simulink model "motorC"  (R2017b)
settings: Solver=FixedStepAuto  StartTime=0.0  StopTime=60  FixedStep=1/fs  RelTol=1e-3
values from neighbouring files (symbols this model uses):
  den = [1 5.1478 5.5483 9]    [script_motor.m]
  denc = [1 0.0078]    [lab3.m]    (also in script_motor.m = conv([1 9.16],[1 9.16]))
  fs = 100    [lab3.m]    (also in script_motor.m; script_tanks.m = 1000)
  num = 180    [script_motor.m]
  numc = 0.0375*[1 0.1625]    [lab3.m]    (also in script_motor.m = 2.31*conv([1 2.73],[1 2.73]))
settings Model: Creator=adgp97  LastModifiedBy=adgp97

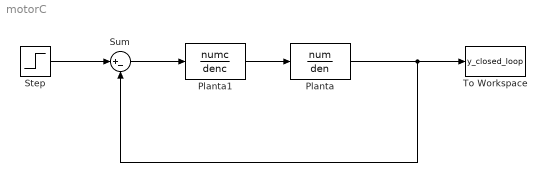
== system motorC ==
  Planta : TransferFcn  Numerator=num  Denominator=den
  Planta1 : TransferFcn  Numerator=numc  Denominator=denc
  Step : Step  Time=30  Before=102  After=112  SampleTime=1/fs
  Sum : Sum  Inputs=|+-
  To Workspace : ToWorkspace  VariableName=y_closed_loop  SampleTime=1/fs
  wires:
  Step/1 -> Sum/1
  Planta/1 -> Sum/2, To Workspace/1
  Planta1/1 -> Planta/1
  Sum/1 -> Planta1/1
